simulink library "libMdl_KalmanFilter"  (R2019b)
settings: Solver=VariableStepAuto  StartTime=0.0  StopTime=10.0  RelTol=1e-3
undefined symbols (not defined in the file): imm_sample_time, P_0, x_0
settings Model: Creator=hwinter  LastModifiedBy=wint_hn
settings DataIOCC: ReturnWorkspaceOutputs=off
settings DebuggingCC: ArithmeticOperatorsInVariantConditions=warning
settings SFSimCC: SimUseLocalCustomCode=off  CustomCodeUndefinedFunction=UseInterfaceOnly
settings RTWCC: RTWUseLocalCustomCode=off

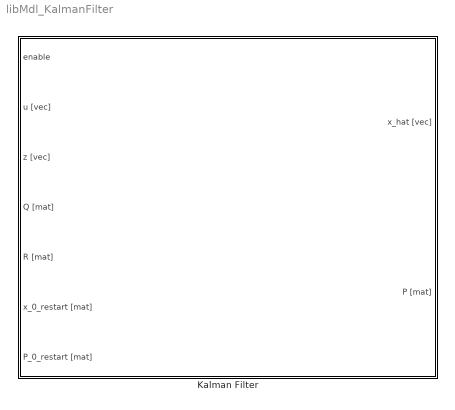
== system libMdl_KalmanFilter ==
  Kalman Filter : Subsystem  mask(Kalman Filter){mv_sample_time=imm_sample_time, mv_x_0=x_0, mv_P_0=P_0, mv_state_transition_function=simFcn_Imm_Trash_StateTransitionFcn, mv_measurement_function=simFcn_Imm_MeasurementFcn, mv_residuum_function=simFcn_Imm_ResiduumFcn}
      mask prompts: mv_sample_time "Sample Time:"; mv_x_0 "Initial State:"; mv_P_0 "Initial Covariance:"; mv_state_transition_function "State Transition Function:"; mv_measurement_function "Measurement Function:"; mv_residuum_function "Residuum Function:"
      mask help:
      | Sample Time:
      | Sample time of the block in seconds
      |
      | Initial State:
      | Initial state in correspondens to the state transition functions
      |
      | Initial Covariance:
      | Initial covariance matrix corresponding to the initial state, defined previously
      |
      | State Transition Function:
      | Name of the state transition function, which has to be defined somewhere in the Matlab workspace
      | (example: stateTransitionFcn)
      |
      | Measurement Function:
      | Name of the measurement function, which has to be defined somewhere in the Matlab workspace
      | (example: measurementFcn)
      mask init:
      | % convert strings to numbers
      | mv_state_transition_function = uint8(mv_state_transition_function);
      | mv_measurement_function = uint8(mv_measurement_function);
      | mv_residuum_function = uint8(mv_residuum_function);
      | 
      | % remove unwanted characteres
      | % spaces --> 32
      | % apostrophe --> 39
      | mv_state_transition_function = mv_state_transition_function(~ismember(mv_state_transition_function,[32 39]));
      | mv_measurement_function = mv_measurement_function(~ismember(mv_measurement_function,[32 39]));
      | mv_residuum_function = mv_residuum_function(~ismember(mv_residuum_function,[32 39]));
      mask Display:
      | str1 = sprintf('\\color{black}{\\bfKalman Filter}\n\n');
      | str2 = sprintf('Sample Time: %0.2f\n\n',mv_sample_time);
      | if length(mv_x_0) <= 3
      |     str3 = sprintf('x_0: %s\n',mat2str(mv_x_0,5));
      | else
      |     str3 = sprintf('x_0: [...]\n');
      | end % if
      | if length(mv_P_0) == 1
      |     str4 = sprintf('P_0: %0.2f\n\n',mv_P_0);
      | else
      |     str4 = sprintf('P_0: [...]\n\n');
      | end % if
      | str5 = sprintf('State Transition Function: {\\it %s} \n',mv_state_transition_function);
      | str6 = sprintf('Measurement Function: {\\it %s} \n',mv_measurement_function);
      | % if isempty(mv_residuum_function)
      | %     str7 = '';
      | % else
      |     str7 = sprintf('Residuum Function: {\\it %s} \n',mv_residuum_function);
      | % end % if
      | str5 = strrep(str5, '_', '\_');
      | str6 = strrep(str6, '_', '\_');
      | str7 = strrep(str7, '_', '\_');
      | 
      | 
      | str = [str1,str2,str3,str4,str5,str6,str7];
      | 
      | text( 0.5,0.5, ...
      |       str, ...
      |       'horizontalAlignment', 'center', ...
      |       'texmode','on' ...
      |     )

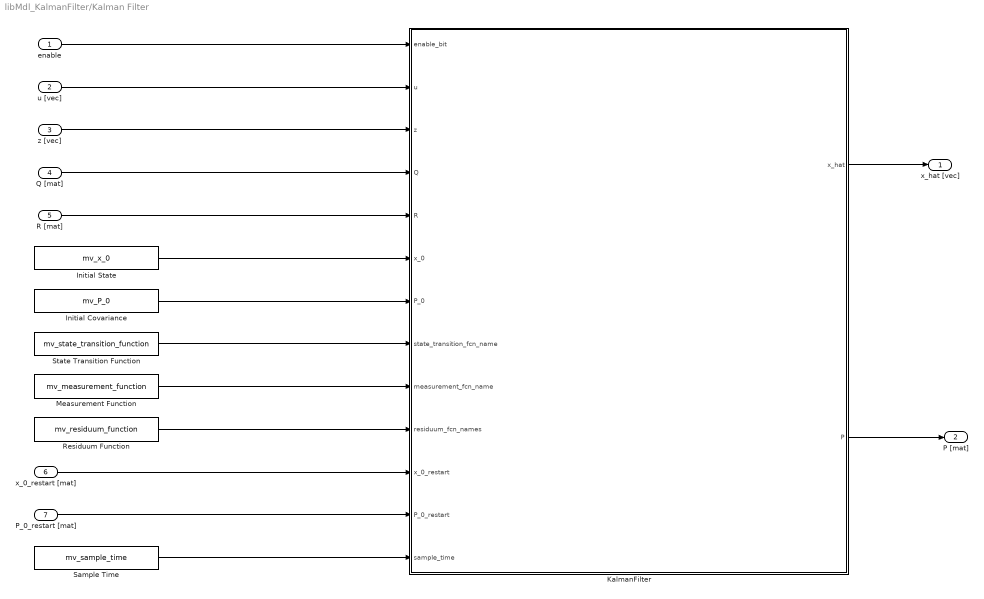
== system libMdl_KalmanFilter/Kalman Filter ==
  enable : Inport
  u [vec] : Inport  Port=2
  z [vec] : Inport  Port=3
  Q [mat] : Inport  Port=4
  R [mat] : Inport  Port=5
  x_0_restart [mat] : Inport  Port=6  SampleTime=mv_sample_time
  P_0_restart [mat] : Inport  Port=7  SampleTime=mv_sample_time
  Initial Covariance : Constant  Value=mv_P_0
  Initial State : Constant  Value=mv_x_0
  KalmanFilter : MATLAB Function  TreatAsAtomicUnit=on  SystemSampleTime=mv_sample_time
  Measurement Function : Constant  Value=mv_measurement_function  VectorParams1D=off
  Residuum Function : Constant  Value=mv_residuum_function
  Sample Time : Constant  Value=mv_sample_time
  State Transition Function : Constant  Value=mv_state_transition_function  VectorParams1D=off
  x_hat [vec] : Outport  VectorParamsAs1DForOutWhenUnconnected=off
  P [mat] : Outport  Port=2  VectorParamsAs1DForOutWhenUnconnected=off
  wires:
  x_0_restart [mat]/1 -> KalmanFilter/11(x_0_restart)
  P_0_restart [mat]/1 -> KalmanFilter/12(P_0_restart)
  Residuum Function/1 -> KalmanFilter/10(residuum_fcn_names)
  enable/1 -> KalmanFilter/1(enable_bit)
  R [mat]/1 -> KalmanFilter/5(R)
  Q [mat]/1 -> KalmanFilter/4(Q)
  z [vec]/1 -> KalmanFilter/3(z)
  u [vec]/1 -> KalmanFilter/2(u)
  KalmanFilter/1(x_hat) -> x_hat [vec]/1
  KalmanFilter/2(P) -> P [mat]/1
  Sample Time/1 -> KalmanFilter/13(sample_time)
  Initial Covariance/1 -> KalmanFilter/7(P_0)
  Initial State/1 -> KalmanFilter/6(x_0)
  State Transition Function/1 -> KalmanFilter/8(state_transition_fcn_name)
  Measurement Function/1 -> KalmanFilter/9(measurement_fcn_name)

== matlab function libMdl_KalmanFilter/Kalman Filter/KalmanFilter ==
  data: enable_bit input; u input; x_hat output; z input; Q input; R input; x_0 input; P_0 input; state_transition_fcn_name input; measurement_fcn_name input; residuum_fcn_names input; x_0_restart input; P_0_restart input; sample_time input; P output
function [x_hat,P] = simFcn_KalmanFilter(enable_bit,u,z,Q,R,x_0,P_0,state_transition_fcn_name,measurement_fcn_name,residuum_fcn_names,x_0_restart,P_0_restart,sample_time)

coder.extrinsic('eval','gcb','get_param');
coder.extrinsic('calcDiscreteKalmanFilter');

x_hat = coder.nullcopy(zeros(size(x_0)));
P = coder.nullcopy(zeros(length(x_0)));

persistent mem_var_x_hat mem_var_P

% Init ____________________________________________________________________

if isempty(mem_var_x_hat)
    mem_var_x_hat = x_0;
    mem_var_P = P_0;
    
    x_hat = mem_var_x_hat;
    P = mem_var_P;    
    
    return
end % if

if ~enable_bit
    x_hat = x_0_restart;
    P = P_0_restart;    
    return
end % if

if -1 == sample_time
    T_temp = get_param(gcb,'CompiledSampleTime');
    T = T_temp(1);
else
    T = sample_time;
end % if

state_transition_fcn_string = char(state_transition_fcn_name(:)');
measurement_fcn_string = char(measurement_fcn_name(:)');
residuum_fcn_string_i = char(residuum_fcn_names(:)');

% Calculations ____________________________________________________________

% Kalman filtering
[x_hat,P,~,~] = calcDiscreteKalmanFilter(u,z,Q,R,mem_var_x_hat,mem_var_P,state_transition_fcn_string,measurement_fcn_string,T,residuum_fcn_string_i);

% Forwarding for next iteration
mem_var_x_hat = x_hat;
mem_var_P = P;

end % function
